simulink model "example_windowShading_SolarGain"  (R2016b)
settings: Solver=ode45  StartTime=0  StopTime=365*24*3600  MaxStep=600  RelTol=1e-3  EnableMultiTasking=on
undefined symbols (not defined in the file): Dreifach, Wärmeschutzglas
libraries: carnot x6
settings Model: Creator=drhf  LastModifiedBy=drhf
settings DataIOCC: LimitDataPoints=on  SaveFormat=Array
settings OptimizationCC: DefaultParameterBehavior=Inlined  LifeSpan=inf
settings DebuggingCC: UnderspecifiedInitializationDetection=Classic  MergeDetectMultiDrivingBlocksExec=none  SolverPrmCheckMsg=warning  SFUnexpectedBacktrackingDiag=warning  SFNoUnconditionalDefaultTransitionDiag=warning  SFExecutionAtInitializationDiag=none
settings HardwareCC: ProdBitPerPointer=32  ProdBitPerSizeT=32  ProdBitPerPtrDiffT=32  ProdLargestAtomicFloat=None  ProdIntDivRoundTo=Undefined  ProdEndianess=Unspecified  ProdWordSize=32  ProdHWDeviceType=32-bit Generic
settings ModelReferenceCC: PropagateSignalLabelsOutOfModel=off
settings GRTTargetCC: TargetLangStandard=C89/C90 (ANSI)  GeneratePreprocessorConditionals=Disable all
settings ConfigComp: CovMetricSettings=dw  CovHtmlReporting=on  CovSaveCumulativeToWorkspaceVar=on  CovSaveSingleToWorkspaceVar=on  CovExternalEMLEnable=off

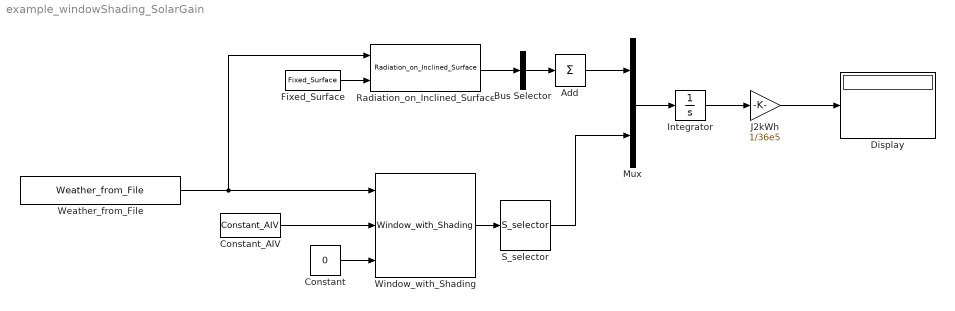
== system example_windowShading_SolarGain ==
  Add : Sum  Inputs=1
  Bus Selector : BusSelector  OutputSignals=Solar_Radiation_direct_surface,Solar_Radiation_diffuse_surface  OutputAsBus=on
  Constant : Constant  Value=0
  Constant_AIV : carnot/Source/Ventilation/Constant_AIV  Tsens=20  Tcon=20  Trad=20  mw=0.012  mco=0.01  rhoair=1.2  cpair=1004  pair=100000  nair=0.5
  Display : Display
  Fixed_Surface : carnot/Weather/Fixed_Surface  colangle=90  colazi=0  colrot=0
  Integrator : Integrator
  J2kWh : Gain  Gain=1/36e5
  Mux : Mux  Inputs=2
  Radiation_on_Inclined_Surface : carnot/Weather/Radiation_on_Inclined_Surface  sky=Perez 1990  reflect=0.2
  S_selector : carnot/Outputs/S_selector  e1=on  e2=off  e3=off  e4=off  e5=off  e6=off  e7=off  e8=off  e9=off  e10=off  e11=off  e12=off  e13=off
  Weather_from_File : carnot/Weather/Weather_from_File  file=DE_TRY2010_04_averageYear  ext=.mat
  Window_with_Shading : carnot/Load/Houses/wall_floor/Window_with_Shading  pos=180  windowsize=[1 1]  frame=0  Ug=1.8  gvalue=0.7  tauzero=0.8  numpanes=2  d=[0.004 0.004]  rho=[2500 2500]  cp="[1008  1008]"  t0=20  misc="[0.2,  0.1,  1,  1]"  shad_type=No shading  type_glazing=Dreifach-Wärmeschutzglas  tau_shad=0.01  bli_a=0.05  bli_b=1  bli_c=0.05  bli_d=0.05  bli_alpha=90  bli_refl=0.2
  wires:
  Constant_AIV/1 -> Window_with_Shading/2
  Weather_from_File/1 -> Radiation_on_Inclined_Surface/1, Window_with_Shading/1
  Constant/1 -> Window_with_Shading/3
  Window_with_Shading/1 -> S_selector/1
  Integrator/1 -> J2kWh/1
  J2kWh/1 -> Display/1
  Fixed_Surface/1 -> Radiation_on_Inclined_Surface/2
  Radiation_on_Inclined_Surface/1 -> Bus Selector/1
  Bus Selector/1 -> Add/1
  S_selector/1 -> Mux/2
  Mux/1 -> Integrator/1
  Add/1 -> Mux/1
